simulink model "sfwb_boost_inverter"  (R2020a)
settings: Solver=VariableStepAuto  StartTime=0.0  StopTime=10.0  RelTol=1e-3
undefined symbols (not defined in the file or in its folder): Ion, Lithium
libraries: powerlib x36, powerlib_meascontrol x3, electricdrivelib x2, re_lib x2, fuzblock x1
settings Model: Creator=Home  LastModifiedBy=Home

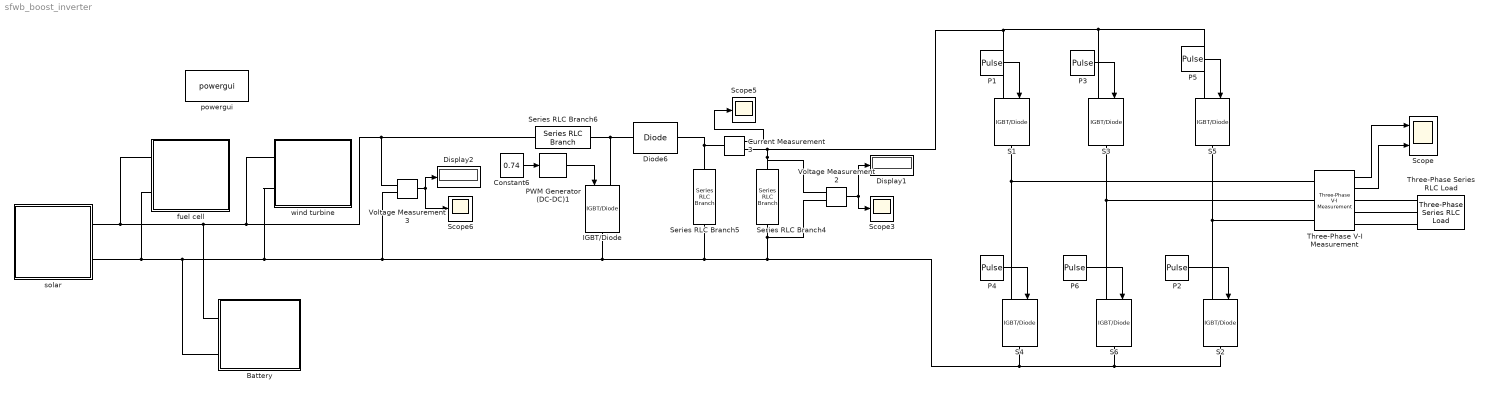
== system sfwb_boost_inverter ==
  Battery : Subsystem
      mask Display: image('C:\Users\Home\Downloads\battery.jpg'); % Use "Edit Image" on toolstrip to change.
  Constant6 : Constant  Value=0.74
  Current Measurement3 : powerlib/Measurements/Current Measurement  PhasorSimulation=off  OutputType=Complex  PSBequivalent=0
  Diode6 : powerlib/Power Electronics/Diode  Ron=0.001  Lon=0  Vf=0.8  IC=0  UseSnubber=off  Rs=500  Cs=250e-9  Measurements=off
  Display1 : Display
  Display2 : Display
  IGBT/Diode : powerlib/Power Electronics/IGBT//Diode  Ron=1e-3  Rs=1e5  Cs=inf  Measurements=off
  "P1 " : DiscretePulseGenerator  PulseType=Time based  Period=0.02  PulseWidth=50  PhaseDelay=0*0.02/360
  P2 : DiscretePulseGenerator  PulseType=Time based  Period=0.02  PulseWidth=50  PhaseDelay=60*0.02/360
  P3 : DiscretePulseGenerator  PulseType=Time based  Period=0.02  PulseWidth=50  PhaseDelay=120*0.02/360
  P4 : DiscretePulseGenerator  PulseType=Time based  Period=0.02  PulseWidth=50  PhaseDelay=180*0.02/360
  P5 : DiscretePulseGenerator  PulseType=Time based  Period=0.02  PulseWidth=50  PhaseDelay=240*0.02/360
  P6 : DiscretePulseGenerator  PulseType=Time based  Period=0.02  PulseWidth=50  PhaseDelay=300*0.02/360
  PWM Generator (DC-DC)1 : powerlib_meascontrol/Pulse & Signal Generators/PWM Generator (DC-DC)  Fsw=5000  Ts=0
  S{1..6} (6 alike) : powerlib/Power Electronics/IGBT//Diode  Ron=1e-3  Rs=1e5  Cs=inf  Measurements=off
  Scope : Scope  NumInputPorts=2
  Scope3 : Scope
  Scope5 : Scope
  Scope6 : Scope
  Series RLC Branch4 : powerlib/Elements/Series RLC Branch  LConnTagsString=__new0  RConnTagsString=__new0  BranchType=R  Resistance=20  Inductance=1e-3  SetiL0=off  InitialCurrent=0  Capacitance=1e-6  Setx0=off  InitialVoltage=0  Measurements=None
  Series RLC Branch5 : powerlib/Elements/Series RLC Branch  LConnTagsString=__new0  RConnTagsString=__new0  BranchType=C  Resistance=1  Inductance=1e-3  SetiL0=off  InitialCurrent=0  Capacitance=145e-6  Setx0=off  InitialVoltage=0  Measurements=None
  Series RLC Branch6 : powerlib/Elements/Series RLC Branch  LConnTagsString=__new0  RConnTagsString=__new0  BranchType=L  Resistance=1  Inductance=66e-6  SetiL0=off  InitialCurrent=0  Capacitance=1e-6  Setx0=off  InitialVoltage=0  Measurements=None
  Three-Phase Series RLC Load : powerlib/Elements/Three-Phase Series RLC Load  LConnTagsString=A|B|C  Configuration=Y (grounded)  NominalVoltage=1000  Vabc=[1e3 1e3 1e3]  Vabcp=[1e3 1e3 1e3]  NominalFrequency=60  UnbalancedPower=off  ActivePower=10e3  InductivePower=100  CapacitivePower=100  Pabc=[10e3 9e3 11e3]  QLabc=[100 90 110]  QCabc=[100 90 110]  Pabcp=[10e3 9e3 11e3]  QLabcp=[100 90 110]  QCabcp=[100 90 110]  Measurements=None  LoadType=constant Z
  Three-Phase V-I Measurement : powerlib/Measurements/Three-Phase V-I Measurement  VoltageMeasurement=phase-to-ground  SetLabelV=off  LabelV=Vabc  Vpu=off  VpuLL=off  CurrentMeasurement=yes  SetLabelI=off  LabelI=Iabc  Ipu=off  Pbase=100e6  Vbase=500e3  OutputType=Complex  PhasorSimulation=off  PSBequivalent=0
  Voltage Measurement2 : powerlib/Measurements/Voltage Measurement  PhasorSimulation=off  OutputType=Complex  PSBequivalent=0
  Voltage Measurement3 : powerlib/Measurements/Voltage Measurement  PhasorSimulation=off  OutputType=Complex  PSBequivalent=0
  fuel cell : Subsystem
      mask Display: image('C:\Users\Home\Downloads\Hydrogen_Oxygen-Fuel-Cell.jpg'); % Use "Edit Image" on toolstrip to change.
  powergui : powerlib/powergui  Priority=1  SimulationMode=Discrete  SampleTime=1e-5  frequency=60  Iterations=50  frequencyindice=0  Pbase=100e6  ErrMax=1e-4  UnitsV=kV  UnitsW=MW  buscounter=0  FunctionMessages=off  echomessages=off  EnableUseOfTLC=off  CurrentSourceSwitches=off  DisableSnubberDevices=off  DisableRonSwitches=off  DisableVfSwitches=off  DisplayEquations=off  AutomaticDiscreteSolvers=off  SolverType=Tustin/Backward Euler (TBE)  Interpol=off  ExternalGateDelay=off  methode=off  Ts=100  x0status=blocks  SPID=on  SwTol=0  HookPort=off  NonlinearTolerance=1e-4  nMaxIteration=100  ContinueOnMaxIteration=off  RestoreLinks=warning  ResistiveCurrentMeasurement=off  Frange=[0:2:500]  Ylog=off  Xlog=on  ShowGrid=off  save=off  variable=ZData  structure=0  ZoomFFT=off  StartTime=0.0  cycles=1  DisplayStyle=1  fundamental=60  FreqAxis=off  MaxFrequency=1000  frequencyindicesteady=1  RmsSteady=1  display=off
  solar : Subsystem
      mask Display: image('C:\Users\Home\Downloads\solar.jpeg'); % Use "Edit Image" on toolstrip to change.
  wind turbine : Subsystem
      mask Display: image('C:\Users\Home\Downloads\wind.jpg'); % Use "Edit Image" on toolstrip to change.
  wires:
  Voltage Measurement3/1 -> Scope6/1, Display2/1
  Voltage Measurement2/1 -> Scope3/1, Display1/1
  Constant6/1 -> PWM Generator (DC-DC)1/1
  Current Measurement3/1 -> Scope5/1
  PWM Generator (DC-DC)1/1 -> IGBT/Diode/1
  P5/1 -> S5/1
  P4/1 -> S4/1
  P6/1 -> S6/1
  "P1 "/1 -> S1/1
  P3/1 -> S3/1
  P2/1 -> S2/1
  Three-Phase V-I Measurement/2 -> Scope/2
  Three-Phase V-I Measurement/1 -> Scope/1
  connections:
  Series RLC Branch6/RConn1 -- IGBT/Diode/LConn1 -- Diode6/LConn1
  Series RLC Branch5/LConn1 -- Diode6/RConn1 -- Current Measurement3/LConn1
  solar/RConn1 -- fuel cell/LConn1 -- Battery/LConn1 -- Voltage Measurement3/LConn1 -- Series RLC Branch6/LConn1 -- wind turbine/LConn1
  S3/LConn1 -- S1/LConn1 -- Current Measurement3/RConn1 -- Voltage Measurement2/LConn1 -- Series RLC Branch4/LConn1 -- S5/LConn1
  S4/RConn1 -- Voltage Measurement2/LConn2 -- Series RLC Branch4/RConn1 -- Series RLC Branch5/RConn1 -- IGBT/Diode/RConn1 -- fuel cell/LConn2 -- solar/RConn2 -- Battery/LConn2 -- wind turbine/LConn2 -- Voltage Measurement3/LConn2 -- S6/RConn1 -- S2/RConn1
  S3/RConn1 -- Three-Phase V-I Measurement/LConn2 -- S6/LConn1
  S1/RConn1 -- Three-Phase V-I Measurement/LConn1 -- S4/LConn1
  S5/RConn1 -- Three-Phase V-I Measurement/LConn3 -- S2/LConn1
  Three-Phase Series RLC Load/LConn1 -- Three-Phase V-I Measurement/RConn1
  Three-Phase Series RLC Load/LConn2 -- Three-Phase V-I Measurement/RConn2
  Three-Phase Series RLC Load/LConn3 -- Three-Phase V-I Measurement/RConn3

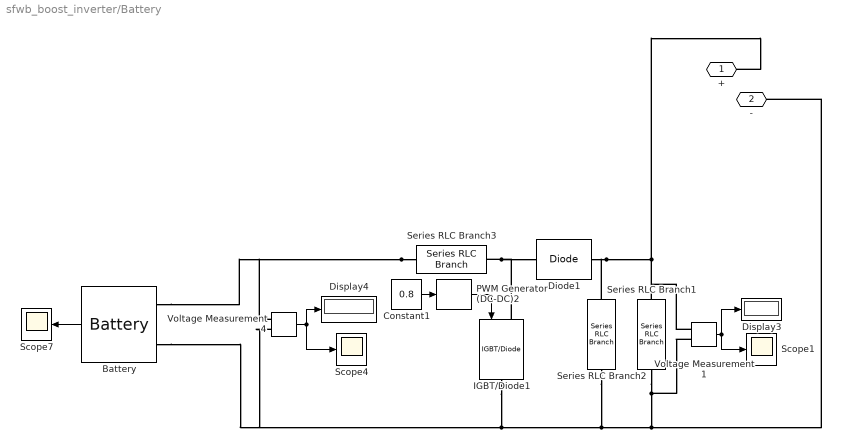
== system sfwb_boost_inverter/Battery ==
  Battery : electricdrivelib/Extra Sources/Battery  BatType=Lithium-Ion  ShowTempParam=off  ThermalPreset=no  ShowAgeParam=off  NomV=7.2  NomQ=5.4  SOC=100  Batt_Tr=30  PresetModel=on  MaxQ=5.4  MinV=5.4  FullV=8.3807  Dis_rate=2.3478  R=0.013333  Normal_OP=4.8835  expZone="[7.7788      0.2653]"  current=[6.5 13 32.5]  Units=Time  Tci=20  NomT=20  T2=-30  MaxQ2=4.8  FullV2=7.1  Normal_OP2=5.655  expZone2="[6.58           1]"  Rca=0.6  ti=2000  Dp=0  Neq0=0  Tsim=1e6  Ta1=25  Qeol=5.4*0.9  Reol=0.013333*1.2  Char_age=[2.3478, 3]  Dis_age=[2.3478, 10]  N1=1500  N2=10500  N3=1000  N4=1400  Ta2=45  N5=950
  Constant1 : Constant  Value=0.8
  Diode1 : powerlib/Power Electronics/Diode  Ron=0.001  Lon=0  Vf=0.8  IC=0  UseSnubber=off  Rs=500  Cs=250e-9  Measurements=off
  Display3 : Display
  Display4 : Display
  IGBT/Diode1 : powerlib/Power Electronics/IGBT//Diode  Ron=1e-3  Rs=1e5  Cs=inf  Measurements=off
  PWM Generator (DC-DC)2 : powerlib_meascontrol/Pulse & Signal Generators/PWM Generator (DC-DC)  Fsw=5000  Ts=0
  Scope1 : Scope
  Scope4 : Scope
  Scope7 : Scope
  Series RLC Branch1 : powerlib/Elements/Series RLC Branch  LConnTagsString=__new0  RConnTagsString=__new0  BranchType=R  Resistance=10  Inductance=1e-3  SetiL0=off  InitialCurrent=0  Capacitance=1e-6  Setx0=off  InitialVoltage=0  Measurements=None
  Series RLC Branch2 : powerlib/Elements/Series RLC Branch  LConnTagsString=__new0  RConnTagsString=__new0  BranchType=C  Resistance=1  Inductance=1e-3  SetiL0=off  InitialCurrent=0  Capacitance=174e-6  Setx0=off  InitialVoltage=0  Measurements=None
  Series RLC Branch3 : powerlib/Elements/Series RLC Branch  LConnTagsString=__new0  RConnTagsString=__new0  BranchType=L  Resistance=1  Inductance=18.37e-6  SetiL0=off  InitialCurrent=0  Capacitance=1e-6  Setx0=off  InitialVoltage=0  Measurements=None
  Voltage Measurement1 : powerlib/Measurements/Voltage Measurement  PhasorSimulation=off  OutputType=Complex  PSBequivalent=0
  Voltage Measurement4 : powerlib/Measurements/Voltage Measurement  PhasorSimulation=off  OutputType=Complex  PSBequivalent=0
  + : PMIOPort  Side=Left
  - : PMIOPort  Port=2  Side=Left
  wires:
  Battery/1 -> Scope7/1
  Voltage Measurement4/1 -> Scope4/1, Display4/1
  Voltage Measurement1/1 -> Scope1/1, Display3/1
  Constant1/1 -> PWM Generator (DC-DC)2/1
  PWM Generator (DC-DC)2/1 -> IGBT/Diode1/1
  connections:
  Voltage Measurement1/LConn2 -- Series RLC Branch1/RConn1 -- -/RConn1 -- Voltage Measurement4/LConn2 -- Battery/LConn2 -- IGBT/Diode1/RConn1 -- Series RLC Branch2/RConn1
  Series RLC Branch3/LConn1 -- Voltage Measurement4/LConn1 -- Battery/LConn1
  Series RLC Branch2/LConn1 -- Diode1/RConn1 -- +/RConn1 -- Voltage Measurement1/LConn1 -- Series RLC Branch1/LConn1
  Series RLC Branch3/RConn1 -- IGBT/Diode1/LConn1 -- Diode1/LConn1

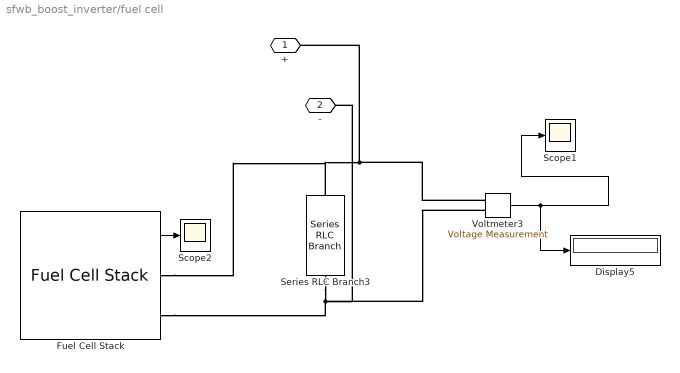
== system sfwb_boost_inverter/fuel cell ==
  Display5 : Display
  Fuel Cell Stack : electricdrivelib/Extra Sources/Fuel Cell Stack  PresetModel=PEMFC - 6 kW - 45 Vdc  FcType=0  Detailed=Detailed  Eoc=[65,63]  NomVI=[133.3,45]  EndVI=[225,37]  Nc=65  n=55  TOp=65  AirFr=300  SuppPress=[1.5,1]  Comp=[99.95,21,1]  SignX=off  SignY=off  FlowRateH2=off  FlowRateAir=off  SystemTemp=off  SystemPH2=off  SystemPAir=off  FCDyn=off  FC_tau=1  Peak_O2=80  V_Under=10
      settings: SourceProductBaseCode=PS
  Scope1 : Scope
  Scope2 : Scope
  Series RLC Branch3 : powerlib/Elements/Series RLC Branch  LConnTagsString=__new0  RConnTagsString=__new0  BranchType=R  Resistance=10  Inductance=1e-3  SetiL0=off  InitialCurrent=0  Capacitance=1e-6  Setx0=off  InitialVoltage=0  Measurements=None
  Voltmeter3 : powerlib/Measurements/Voltage Measurement  PhasorSimulation=off  OutputType=Complex  PSBequivalent=0
  + : PMIOPort  Side=Left
  - : PMIOPort  Port=2  Side=Left
  wires:
  Voltmeter3/1 -> Scope1/1, Display5/1
  Fuel Cell Stack/1 -> Scope2/1
  connections:
  Voltmeter3/LConn1 -- Fuel Cell Stack/RConn1 -- Series RLC Branch3/LConn1 -- +/RConn1
  Fuel Cell Stack/RConn2 -- Series RLC Branch3/RConn1 -- -/RConn1 -- Voltmeter3/LConn2

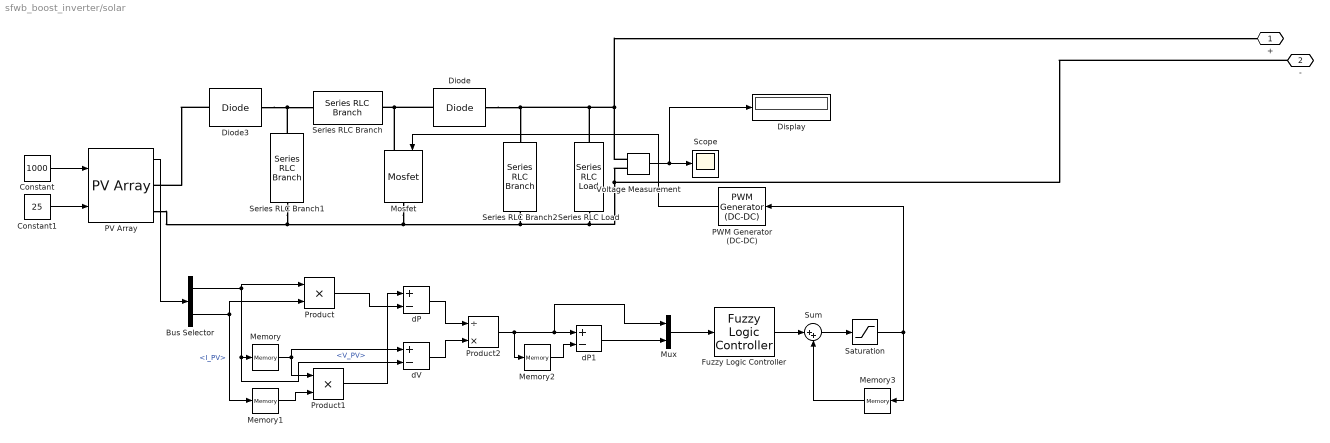
== system sfwb_boost_inverter/solar ==
  Bus Selector : BusSelector  OutputSignals=V_PV,I_PV
  Constant : Constant  Value=1000
  Constant1 : Constant  Value=25
  Diode : powerlib/Power Electronics/Diode  Ron=0.001  Lon=0  Vf=0.8  IC=0  UseSnubber=0  Rs=500  Cs=250e-9  Measurements=off
  Diode3 : powerlib/Power Electronics/Diode  Ron=0.001  Lon=0  Vf=0.8  IC=0  UseSnubber=0  Rs=500  Cs=250e-9  Measurements=off
  Display : Display
  Fuzzy Logic Controller : fuzblock/Fuzzy Logic  Controller  FIS='tipper.fis'  OutputSampleNumber=101  DataType=double  FuzzifiedInputs=off  RuleFiringStrengths=off  RuleOutputs=off  AggregatedOutputs=off  SimulateUsing=Interpreted execution  OutOfRangeInputValueMessage=warning  NoRuleFiredMessage=warning  EmptyOutputFuzzySetMessage=warning
  Memory{,1..3} (4 alike) : Memory
  Mosfet : powerlib/Power Electronics/Mosfet  Ron=0.1  Lon=0  Rd=0.01  Vfd=0  IC=0  Rs=1e5  Cs=inf  Measurements=off
  Mux : Mux  Inputs=2
  PV Array : re_lib/Solar/PV Array  Npar=3  Nser=3  PlotType=one module @ 25 deg.C & specified irradiances  S_vec=[800 ]  Temp_C_vec="[ 45 25  ]"  ModuleName=Kyocera Solar KC200GT  PlotWhenSelected=off  Pm=200.143  Ncell=54  Voc=32.9  Isc=8.21  Vm=26.3  Im=7.61  beta_Voc_pc=-0.35502  alpha_Isc_pc=0.06  beta_Voc=-0.1168  alpha_Isc=0.004926  IL=8.2288  I0=2.3246e-10  nI=0.97736  Rsh=150.6921  Rs=0.34483  RobustModel=off  RobustCellTemperature=25  BAL=on  Tc=1e-6  Tfilter=5e-5
  PWM Generator (DC-DC) : powerlib_meascontrol/Pulse & Signal Generators/PWM Generator (DC-DC)  Fsw=5000  Ts=0
  Product : Product
  Product1 : Product
  Product2 : Product  Inputs=/*
  Saturation : Saturate
  Scope : Scope
  Series RLC Branch : powerlib/Elements/Series RLC Branch  LConnTagsString=__new0  RConnTagsString=__new0  BranchType=L  Resistance=1  Inductance=1e-4  SetiL0=off  InitialCurrent=0  Capacitance=1e-6  Setx0=off  InitialVoltage=0  Measurements=None
  Series RLC Branch1 : powerlib/Elements/Series RLC Branch  LConnTagsString=__new0  RConnTagsString=__new0  BranchType=C  Resistance=1  Inductance=1e-4  SetiL0=off  InitialCurrent=0  Capacitance=4000e-6  Setx0=off  InitialVoltage=0  Measurements=None
  Series RLC Branch2 : powerlib/Elements/Series RLC Branch  LConnTagsString=__new0  RConnTagsString=__new0  BranchType=C  Resistance=1  Inductance=1e-4  SetiL0=off  InitialCurrent=0  Capacitance=50e-6  Setx0=off  InitialVoltage=0  Measurements=None
  Series RLC Load : powerlib/Elements/Series RLC Load  LConnTagsString=a  RConnTagsString=__new0  NominalVoltage=30  NominalFrequency=50  ActivePower=120  InductivePower=0  CapacitivePower=0  Setx0=off  InitialVoltage=0  SetiL0=off  InitialCurrent=0  Measurements=None  LoadType=constant Z
  Sum : Sum  Inputs=|++
  Voltage Measurement : powerlib/Measurements/Voltage Measurement  PhasorSimulation=off  OutputType=Complex  PSBequivalent=0
  dP : Sum  Inputs=+-
  dP1 : Sum  Inputs=+-
  dV : Sum  Inputs=+-
  + : PMIOPort  Side=Right
  - : PMIOPort  Port=2  Side=Right
  wires:
  Product2/1 -> Memory2/1, Mux/1, dP1/1
  PWM Generator (DC-DC)/1 -> Mosfet/1
  Fuzzy Logic Controller/1 -> Sum/1
  Mux/1 -> Fuzzy Logic Controller/1
  Memory3/1 -> Sum/2
  Memory/1 -> dV/1, Product1/1
  Saturation/1 -> Memory3/1, PWM Generator (DC-DC)/1
  Bus Selector/2 -> Product/2, Memory1/1  "<I_PV>"
  Memory1/1 -> Product1/2
  PV Array/1 -> Bus Selector/1
  Voltage Measurement/1 -> Display/1, Scope/1
  Constant1/1 -> PV Array/2
  Memory2/1 -> dP1/2
  dV/1 -> Product2/2
  Bus Selector/1 -> Product/1, dV/2, Memory/1  "<V_PV>"
  dP/1 -> Product2/1
  Product1/1 -> dP/1
  Sum/1 -> Saturation/1
  Constant/1 -> PV Array/1
  Product/1 -> dP/2
  dP1/1 -> Mux/2
  connections:
  Series RLC Branch1/RConn1 -- PV Array/RConn2 -- Mosfet/RConn1 -- Series RLC Branch2/RConn1 -- -/RConn1 -- Voltage Measurement/LConn2 -- Series RLC Load/RConn1
  Voltage Measurement/LConn1 -- +/RConn1 -- Diode/RConn1 -- Series RLC Branch2/LConn1 -- Series RLC Load/LConn1
  Diode3/RConn1 -- Series RLC Branch1/LConn1 -- Series RLC Branch/LConn1
  Series RLC Branch/RConn1 -- Mosfet/LConn1 -- Diode/LConn1
  Diode3/LConn1 -- PV Array/RConn1

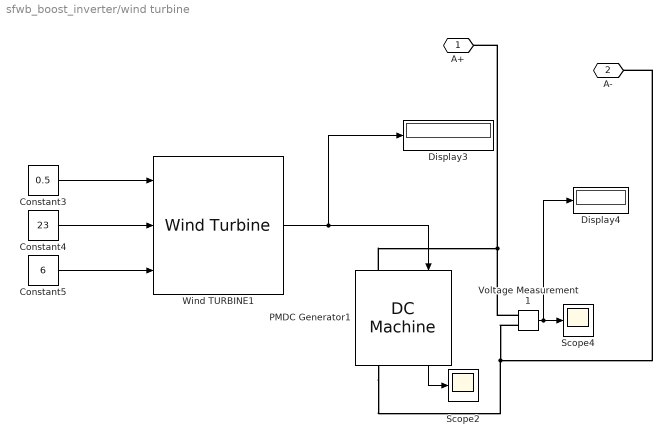
== system sfwb_boost_inverter/wind turbine ==
  Constant3 : Constant  Value=0.5
  Constant4 : Constant  Value=23
  Constant5 : Constant  Value=6
  Display3 : Display
  Display4 : Display
  PMDC Generator1 : powerlib/Machines/DC Machine  PresetModel=No  MechanicalLoad=Torque TL  FieldType=Permanent magnet  ShowDetailedParameters=on  MeasurementBus=off  RLa="[ 0.78  0.016]"  RLf="[ 240  120]"  Laf=1.8  MachineConstant=Torque constant (N.m/A)  Ke=1.8  Kt=1.8  J=0.01  Bm=0.09  Tf=0  w0=1  Ifinit=1  TsPowergui=0  TsBlock=-1
  Scope2 : Scope
  Scope4 : Scope
  Voltage Measurement1 : powerlib/Measurements/Voltage Measurement  PhasorSimulation=off  OutputType=Complex  PSBequivalent=0
  Wind TURBINE1 : re_lib/Wind Generation/Wind Turbine  Pnom=120  Pelec_base=120/0.9  wind_base=2.51  P_wind_base=0.73  speed_nom=0.6  pitch_angle=0  c1_c6="[0.51763          116          0.4            5           21     0.006795]"  cp_nom=0.48  lambda_nom=8.1
      settings: SourceProductBaseCode=PS
  A+ : PMIOPort  Side=Left
  A- : PMIOPort  Port=2  Side=Left
  wires:
  Wind TURBINE1/1 -> Display3/1, PMDC Generator1/1
  Constant3/1 -> Wind TURBINE1/1
  Constant4/1 -> Wind TURBINE1/2
  Constant5/1 -> Wind TURBINE1/3
  PMDC Generator1/1 -> Scope2/1
  Voltage Measurement1/1 -> Display4/1, Scope4/1
  connections:
  Voltage Measurement1/LConn1 -- A+/RConn1 -- PMDC Generator1/LConn1
  Voltage Measurement1/LConn2 -- PMDC Generator1/RConn1 -- A-/RConn1
